simulink model "stateSpaceEigenTest_discrete"  (R2013b)
settings: Solver=FixedStepDiscrete  StartTime=0.0  StopTime=10  FixedStep=0.001  RelTol=1e-3
InitFcn:
  | dimX = 40;
  | dimU = 42;
  | dimY = 42;
  | 
  | Ts = 1/100;
  | 
  | n = dimX; % choose the size
  | d = diag(-rand(1,n)); % create the eigenvalues
  | v = randn(n,n); % create the eigenvectors
  | % be sure they are normalized (but they don't have to be)
  | for ind = 1:n
  |     v(:,n) = v(:,n)/mean(v(:,n));
  | end
  | % Construct x, the matrix with negative eigenvalues
  | matA = v*d*v'; % has negative eigenvalues
  | 
  | % matA = rand(dimX,dimX);
  |     matB = rand(dimX,dimU);
  |     matC = rand(dimU,dimX);
  |     matD = rand(dimY,dimY);
  | 
  | sys=c2d(ss(matA,matB,matC,matD),Ts);
  | matA = sys.A;
  | matB = sys.B;
  | matC = sys.C;
  | matD = sys.D;
  | 
  | vect_x0 = zeros(dimX,1);
  | 
  | disp( sprintf('\ndimension to test is dim = %i',dimX) )
StopFcn:
  | disp('');
  | len = size(original.Data);
  | valid = 1;
  | 
  | biggestError = 0;
  | 
  | for k=1:dimY
  |     t = original.Data(k,1,:);
  |     temp = reshape(t,length(t),1);
  |     temp1 = abs( temp - own.Data(:,k)) > 1e-10;
  |     tt =  max(abs(temp - own.Data(:,k)));
  | 
  |     if( tt > biggestError )
  |         biggestError = tt;
  |     end
  | end
  | 
  | if( any( temp1 ) )
  |   error('mismatch during comparison')
  |   valid = 0;
  | end
  | 
  | if( valid == 1 )
  |   disp('no mismatch found!')
  |   disp( sprintf('greatest deviation is %f*1e-13', biggestError*1e13) )
  | end
settings Model: Creator=rtai-ao  LastModifiedBy=rtai-ao
settings RTWCC: SystemTargetFile=rtai.tlc  TemplateMakefile=rtai.tmf  Description=Linux RTAI Real-Time Target  GenerateReport=on  ProcessScript=rtai_make_rtw_hook  BuildConfiguration=Faster Runs
settings STFCustomTargetCC: ModelReferenceCompliant=off  GeneratePreprocessorConditionals=Disable all  MatFileLogging=on  MATLABClassNameForMDSCustomization=Simulink.SoftwareTarget.TargetSpecificTriggerConfigurationBase  SystemTargetFile=rtai.tlc

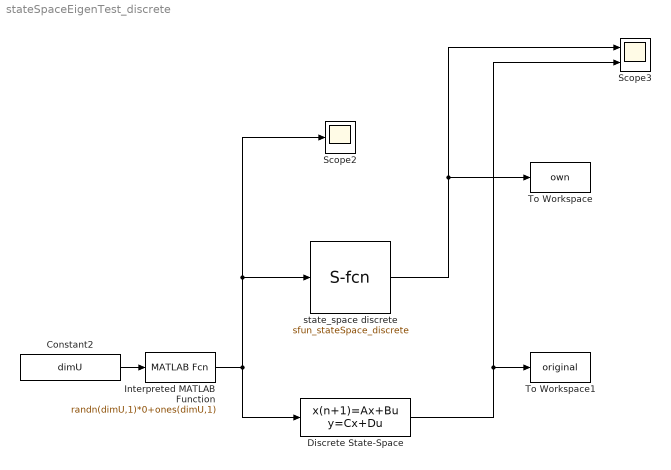
== system stateSpaceEigenTest_discrete ==
  Constant2 : Constant  Value=dimU  VectorParams1D=off
  Discrete State-Space : DiscreteStateSpace  A=matA  B=matB  C=matC  D=matD  X0=vect_x0  SampleTime=Ts
  Interpreted MATLAB Function : MATLABFcn  MATLABFcn=randn(dimU,1)*0+ones(dimU,1)  Output1D=off
  Scope2 : Scope
  Scope3 : Scope  NumInputPorts=2
      settings: YMin=-5~-5  YMax=5~5  SaveName=ScopeData2
  To Workspace : ToWorkspace  VariableName=own  SampleTime=-1  SaveFormat=Timeseries
  To Workspace1 : ToWorkspace  VariableName=original  SampleTime=-1  SaveFormat=Timeseries
  state_space discrete : S-Function  FunctionName=sfun_stateSpace_discrete  Parameters=matrixA,matrixB,matrixC,matrixD,x0,sampleTime  EnableBusSupport=off  mask{matrixA=matA, matrixB=matB, matrixC=matC, matrixD=matD, x0=vect_x0, sampleTime=Ts}
      mask prompts: matrixA "Matrix A"; matrixB "Matrix B"; matrixC "Matrix C"; matrixD "Matrix D"; x0 "initial value (x0)"; sampleTime "Sample Time"
      mask Display: image('state_space_discrete.png')
  wires:
  Interpreted MATLAB Function/1 -> Discrete State-Space/1, Scope2/1, state_space discrete/1
  Constant2/1 -> Interpreted MATLAB Function/1
  Discrete State-Space/1 -> Scope3/2, To Workspace1/1
  state_space discrete/1 -> Scope3/1, To Workspace/1
